simulink model "nonlinear_inverted_pendulum"  (R2025a)
settings: Solver=FixedStepAuto  StartTime=0.0  StopTime=10.0  RelTol=1e-3
undefined symbols (not defined in the file): dth1_0, dth2_0, dxc_0, th1_0, th2_0, xc_0
settings Model: Creator=amoralesma  LastModifiedBy=amoralesma

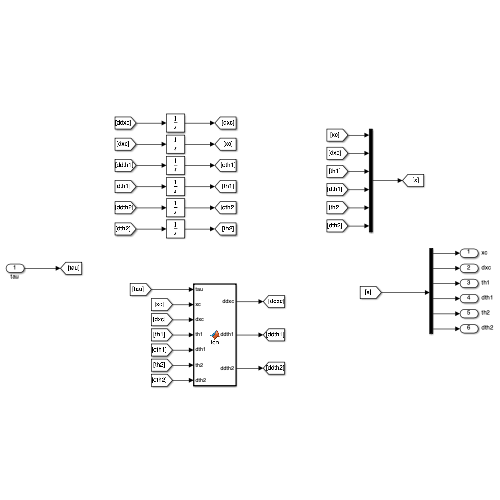
[thumbnail: Simulink's stored preview of the top-level diagram]
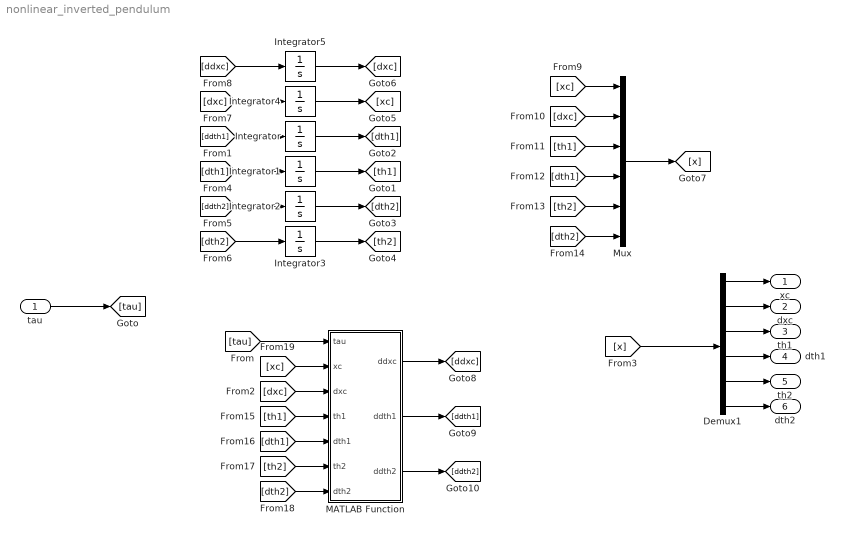
== system nonlinear_inverted_pendulum ==
  tau : Inport
  Demux1 : Demux  Outputs=6
  Integrator : Integrator  InitialCondition=dth1_0
  Integrator1 : Integrator  InitialCondition=th1_0
  Integrator2 : Integrator  InitialCondition=dth2_0
  Integrator3 : Integrator  InitialCondition=th2_0
  Integrator4 : Integrator  InitialCondition=xc_0
  Integrator5 : Integrator  InitialCondition=dxc_0
  MATLAB Function : MATLAB Function  TreatAsAtomicUnit=on
  Mux : Mux  Inputs=6
  xc : Outport
  dxc : Outport  Port=2
  th1 : Outport  Port=3
  dth1 : Outport  Port=4
  th2 : Outport  Port=5
  dth2 : Outport  Port=6
  wires:
  [th2] -> MATLAB Function/6(th2)
  [ddxc] -> Integrator5/1
  [th1] -> MATLAB Function/4(th1)
  [xc] -> Mux/1
  [tau] -> MATLAB Function/1(tau)
  Integrator/1 -> [dth1]
  Demux1/3 -> th1/1
  Demux1/1 -> xc/1
  [ddth2] -> Integrator2/1
  Integrator3/1 -> [th2]
  Integrator2/1 -> [dth2]
  MATLAB Function/3(ddth2) -> [ddth2]
  Demux1/2 -> dxc/1
  Demux1/5 -> th2/1
  [th2] -> Mux/5
  [x] -> Demux1/1
  Mux/1 -> [x]
  [dth1] -> Mux/4
  [dxc] -> MATLAB Function/3(dxc)
  Integrator5/1 -> [dxc]
  tau/1 -> [tau]
  Integrator1/1 -> [th1]
  [dxc] -> Mux/2
  [dth1] -> MATLAB Function/5(dth1)
  [ddth1] -> Integrator/1
  [dth1] -> Integrator1/1
  MATLAB Function/2(ddth1) -> [ddth1]
  Demux1/4 -> dth1/1
  [dth2] -> MATLAB Function/7(dth2)
  Integrator4/1 -> [xc]
  [xc] -> MATLAB Function/2(xc)
  [dth2] -> Mux/6
  [dxc] -> Integrator4/1
  [dth2] -> Integrator3/1
  MATLAB Function/1(ddxc) -> [ddxc]
  [th1] -> Mux/3
  Demux1/6 -> dth2/1

== matlab function nonlinear_inverted_pendulum/MATLAB Function ==
  data: tau input; xc input; dxc input; ddxc output; th1 input; dth1 input; th2 input; dth2 input; ddth1 output; ddth2 output; parameters parameter
function [ddxc, ddth1, ddth2] = fcn(tau,xc, dxc, th1, dth1, th2, dth2, parameters)

% Parameters 
Mc = parameters.Mc;
m1 = parameters.m1; 
m2 = parameters.m2; 
l1 = parameters.l1; 
l2 = parameters.l2;
g = parameters.g;


ddxc  = (l1*m1*sin(th1)*dth1^2 + l2*m2*sin(th2)*dth2^2 + tau - g*m1*cos(th1)*sin(th1) - g*m2*cos(th2)*sin(th2))/(- m1*cos(th1)^2 - m2*cos(th2)^2 + Mc + m1 + m2);
ddth1 = -(l1*m1*cos(th1)*sin(th1)*dth1^2 + l2*m2*cos(th1)*sin(th2)*dth2^2 + g*m2*sin(th1)*cos(th2)^2 - g*m2*cos(th1)*sin(th2)*cos(th2) + tau*cos(th1) - g*m1*sin(th1) - g*m2*sin(th1) - Mc*g*sin(th1))/(l1*(- m1*cos(th1)^2 - m2*cos(th2)^2 + Mc + m1 + m2));
ddth2 = -(l1*m1*cos(th2)*sin(th1)*dth1^2 + l2*m2*cos(th2)*sin(th2)*dth2^2 + g*m1*sin(th2)*cos(th1)^2 - g*m1*cos(th2)*sin(th1)*cos(th1) + tau*cos(th2) - g*m1*sin(th2) - g*m2*sin(th2) - Mc*g*sin(th2))/(l2*(- m1*cos(th1)^2 - m2*cos(th2)^2 + Mc + m1 + m2));
